simulink model "case9"  (R2024b)
settings: Solver=FixedStepAuto  StartTime=0  StopTime=1  FixedStep=1e-7  RelTol=1e-3
values from neighbouring files (symbols this model uses):
  SG_D_1_D = 0.01056    [IEEE9_case_parameters.m]    (also in case1_parameters.m; case2_parameters.m; case3_parameters.m; case4_parameters.m)
  SG_D_1_EnableSaturation = 0    [IEEE9_case_parameters.m]    (also in case1_parameters.m; case2_parameters.m; case3_parameters.m; case4_parameters.m)
  SG_D_1_f0 = 60    [IEEE9_case_parameters.m]    (also in case1_parameters.m; case2_parameters.m; case3_parameters.m; case4_parameters.m)
  SG_D_1_H = 7.5    [IEEE9_case_parameters.m]    (also in case1_parameters.m; case2_parameters.m; case3_parameters.m; case4_parameters.m)
  SG_D_1_K_A = 20    [IEEE9_case_parameters.m]    (also in case1_parameters.m; case2_parameters.m; case3_parameters.m; case4_parameters.m)
  SG_D_1_K_E = 1.000000e+1    (= 10)    [IEEE9_case_parameters.m]    (also in case1_parameters.m; case2_parameters.m; case3_parameters.m; case4_parameters.m)
  SG_D_1_K_F = 2.363    [IEEE9_case_parameters.m]    (also in case1_parameters.m; case2_parameters.m; case3_parameters.m; case4_parameters.m)
  SG_D_1_K_s = 0.5    [IEEE9_case_parameters.m]    (also in case1_parameters.m = 5; case2_parameters.m = 5; case3_parameters.m = 5; case4_parameters.m = 5)
  SG_D_1_R_a = 0.001088    [IEEE9_case_parameters.m]    (also in case1_parameters.m; case2_parameters.m; case3_parameters.m; case4_parameters.m)
  SG_D_1_S_A = 1    [IEEE9_case_parameters.m]    (also in case1_parameters.m; case2_parameters.m; case3_parameters.m; case4_parameters.m)
  SG_D_1_S_B = 0.103    [IEEE9_case_parameters.m]    (also in case1_parameters.m; case2_parameters.m; case3_parameters.m; case4_parameters.m)
  SG_D_1_S_N = 10.659857    [IEEE9_case_parameters.m]    (also in case1_parameters.m; case2_parameters.m; case3_parameters.m; case4_parameters.m)
  SG_D_1_SpeedPara = 200    [IEEE9_case_parameters.m]    (also in case1_parameters.m; case2_parameters.m; case3_parameters.m; case4_parameters.m)
  SG_D_1_T_0 = 0.720173    [IEEE9_case_parameters.m]    (also in case1_parameters.m = 0.755522; case2_parameters.m = 0.808931; case3_parameters.m = 0.869402; case4_parameters.m = 0.729316)
  SG_D_1_T_1 = 0.3    [IEEE9_case_parameters.m]    (also in case1_parameters.m; case2_parameters.m; case3_parameters.m; case4_parameters.m)
  SG_D_1_T_2 = 0.05    [IEEE9_case_parameters.m]    (also in case1_parameters.m; case2_parameters.m; case3_parameters.m; case4_parameters.m)
  SG_D_1_T_3 = 0.02    [IEEE9_case_parameters.m]    (also in case1_parameters.m; case2_parameters.m; case3_parameters.m; case4_parameters.m)
  SG_D_1_T_4 = 0.005    [IEEE9_case_parameters.m]    (also in case1_parameters.m; case2_parameters.m; case3_parameters.m; case4_parameters.m)
  SG_D_1_T_A = 0.02    [IEEE9_case_parameters.m]    (also in case1_parameters.m; case2_parameters.m; case3_parameters.m; case4_parameters.m)
  SG_D_1_T_dd = 8.000000e+0    (= 8)    [IEEE9_case_parameters.m]    (also in case1_parameters.m; case2_parameters.m; case3_parameters.m; case4_parameters.m)
  SG_D_1_T_ddd = 0.04    [IEEE9_case_parameters.m]    (also in case1_parameters.m; case2_parameters.m; case3_parameters.m; case4_parameters.m)
  SG_D_1_T_E = 0.314    [IEEE9_case_parameters.m]    (also in case1_parameters.m; case2_parameters.m; case3_parameters.m; case4_parameters.m)
  SG_D_1_T_F = 0.35    [IEEE9_case_parameters.m]    (also in case1_parameters.m; case2_parameters.m; case3_parameters.m; case4_parameters.m)
  SG_D_1_T_qd = 0.8    [IEEE9_case_parameters.m]    (also in case1_parameters.m; case2_parameters.m; case3_parameters.m; case4_parameters.m)
  SG_D_1_T_qdd = 0.02    [IEEE9_case_parameters.m]    (also in case1_parameters.m; case2_parameters.m; case3_parameters.m; case4_parameters.m)
  SG_D_1_T_speed = 0.1    [IEEE9_case_parameters.m]    (also in case1_parameters.m = 200; case2_parameters.m = 200; case3_parameters.m = 200; case4_parameters.m = 200)
  SG_D_1_T_w = 0.5    [IEEE9_case_parameters.m]    (also in case1_parameters.m; case2_parameters.m; case3_parameters.m; case4_parameters.m)
  SG_D_1_V_ref = 1.990276    [IEEE9_case_parameters.m]    (also in case1_parameters.m = 2.042296; case2_parameters.m = 2.051388; case3_parameters.m = 2.089584; case4_parameters.m = 2.01845)
  SG_D_1_w_ref = 376.991118    [IEEE9_case_parameters.m]    (also in case1_parameters.m; case2_parameters.m; case3_parameters.m; case4_parameters.m)
  SG_D_1_wb = 6.000000e+1    (= 60)    [IEEE9_case_parameters.m]    (also in case1_parameters.m; case2_parameters.m; case3_parameters.m; case4_parameters.m)
  SG_D_1_x_d = 1.9    [IEEE9_case_parameters.m]    (also in case1_parameters.m; case2_parameters.m; case3_parameters.m; case4_parameters.m)
  SG_D_1_x_dd = 0.302    [IEEE9_case_parameters.m]    (also in case1_parameters.m; case2_parameters.m; case3_parameters.m; case4_parameters.m)
  SG_D_1_x_ddd = 0.204    [IEEE9_case_parameters.m]    (also in case1_parameters.m; case2_parameters.m; case3_parameters.m; case4_parameters.m)
  SG_D_1_x_l = 0.05    [IEEE9_case_parameters.m]    (also in case1_parameters.m; case2_parameters.m; case3_parameters.m; case4_parameters.m)
  SG_D_1_x_q = 1.3    [IEEE9_case_parameters.m]    (also in case1_parameters.m; case2_parameters.m; case3_parameters.m; case4_parameters.m)
  SG_D_1_x_qd = 0.5    [IEEE9_case_parameters.m]    (also in case1_parameters.m; case2_parameters.m; case3_parameters.m; case4_parameters.m)
  SG_D_1_x_qdd = 0.3    [IEEE9_case_parameters.m]    (also in case1_parameters.m; case2_parameters.m; case3_parameters.m; case4_parameters.m)
  SG_D_2_D = 0.02    [IEEE9_case_parameters.m]    (also in case1_parameters.m; case2_parameters.m; case3_parameters.m; case4_parameters.m)
  SG_D_2_EnableSaturation = 0    [IEEE9_case_parameters.m]    (also in case1_parameters.m; case2_parameters.m; case3_parameters.m; case4_parameters.m)
  SG_D_2_f0 = 60    [IEEE9_case_parameters.m]    (also in case1_parameters.m; case2_parameters.m; case3_parameters.m; case4_parameters.m)
  SG_D_2_H = 8.000000e+0    (= 8)    [IEEE9_case_parameters.m]    (also in case1_parameters.m; case2_parameters.m; case3_parameters.m; case4_parameters.m)
  SG_D_2_K_A = 20    [IEEE9_case_parameters.m]    (also in case1_parameters.m; case2_parameters.m; case3_parameters.m; case4_parameters.m)
  SG_D_2_K_E = 1.000000e+1    (= 10)    [IEEE9_case_parameters.m]    (also in case1_parameters.m; case2_parameters.m; case3_parameters.m; case4_parameters.m)
  SG_D_2_K_F = 2.363    [IEEE9_case_parameters.m]    (also in case1_parameters.m; case2_parameters.m; case3_parameters.m; case4_parameters.m)
  SG_D_2_K_s = 0.5    [IEEE9_case_parameters.m]    (also in case1_parameters.m = 4; case2_parameters.m = 4; case3_parameters.m = 4; case4_parameters.m = 4)
  SG_D_2_R_a = 0.001088    [IEEE9_case_parameters.m]    (also in case1_parameters.m; case2_parameters.m; case3_parameters.m; case4_parameters.m)
  SG_D_2_S_A = 1    [IEEE9_case_parameters.m]    (also in case1_parameters.m; case2_parameters.m; case3_parameters.m; case4_parameters.m)
  SG_D_2_S_B = 0.103    [IEEE9_case_parameters.m]    (also in case1_parameters.m; case2_parameters.m; case3_parameters.m; case4_parameters.m)
  SG_D_2_S_N = 10.659857    [IEEE9_case_parameters.m]    (also in case1_parameters.m; case2_parameters.m; case3_parameters.m; case4_parameters.m)
  SG_D_2_SpeedPara = 200    [IEEE9_case_parameters.m]    (also in case1_parameters.m; case2_parameters.m; case3_parameters.m; case4_parameters.m)
  SG_D_2_T_0 = 1.632913    [IEEE9_case_parameters.m]    (also in case1_parameters.m = 1.632925; case2_parameters.m = 1.632915; case3_parameters.m = 1.632914; case4_parameters.m = 1.632927)
  SG_D_2_T_1 = 0.2    [IEEE9_case_parameters.m]    (also in case1_parameters.m; case2_parameters.m; case3_parameters.m; case4_parameters.m)
  SG_D_2_T_2 = 0.05    [IEEE9_case_parameters.m]    (also in case1_parameters.m; case2_parameters.m; case3_parameters.m; case4_parameters.m)
  SG_D_2_T_3 = 0.02    [IEEE9_case_parameters.m]    (also in case1_parameters.m; case2_parameters.m; case3_parameters.m; case4_parameters.m)
  SG_D_2_T_4 = 0.005    [IEEE9_case_parameters.m]    (also in case1_parameters.m; case2_parameters.m; case3_parameters.m; case4_parameters.m)
  SG_D_2_T_A = 0.02    [IEEE9_case_parameters.m]    (also in case1_parameters.m; case2_parameters.m; case3_parameters.m; case4_parameters.m)
  SG_D_2_T_dd = 7.9    [IEEE9_case_parameters.m]    (also in case1_parameters.m; case2_parameters.m; case3_parameters.m; case4_parameters.m)
  SG_D_2_T_ddd = 0.04    [IEEE9_case_parameters.m]    (also in case1_parameters.m; case2_parameters.m; case3_parameters.m; case4_parameters.m)
  SG_D_2_T_E = 0.314    [IEEE9_case_parameters.m]    (also in case1_parameters.m; case2_parameters.m; case3_parameters.m; case4_parameters.m)
  SG_D_2_T_F = 0.35    [IEEE9_case_parameters.m]    (also in case1_parameters.m; case2_parameters.m; case3_parameters.m; case4_parameters.m)
  SG_D_2_T_qd = 0.8    [IEEE9_case_parameters.m]    (also in case1_parameters.m; case2_parameters.m; case3_parameters.m; case4_parameters.m)
  SG_D_2_T_qdd = 0.015    [IEEE9_case_parameters.m]    (also in case1_parameters.m; case2_parameters.m; case3_parameters.m; case4_parameters.m)
  SG_D_2_T_speed = 0.1    [IEEE9_case_parameters.m]    (also in case1_parameters.m = 150; case2_parameters.m = 150; case3_parameters.m = 150; case4_parameters.m = 150)
  SG_D_2_T_w = 0.35    [IEEE9_case_parameters.m]    (also in case1_parameters.m; case2_parameters.m; case3_parameters.m; case4_parameters.m)
  SG_D_2_V_ref = 2.58547    [IEEE9_case_parameters.m]    (also in case1_parameters.m = 2.597896; case2_parameters.m = 2.587136; case3_parameters.m = 2.586042; case4_parameters.m = 2.599679)
  SG_D_2_w_ref = 376.991118    [IEEE9_case_parameters.m]    (also in case1_parameters.m; case2_parameters.m; case3_parameters.m; case4_parameters.m)
  SG_D_2_wb = 6.000000e+1    (= 60)    [IEEE9_case_parameters.m]    (also in case1_parameters.m; case2_parameters.m; case3_parameters.m; case4_parameters.m)
  SG_D_2_x_d = 1.8    [IEEE9_case_parameters.m]    (also in case1_parameters.m; case2_parameters.m; case3_parameters.m; case4_parameters.m)
  SG_D_2_x_dd = 0.302    [IEEE9_case_parameters.m]    (also in case1_parameters.m; case2_parameters.m; case3_parameters.m; case4_parameters.m)
  SG_D_2_x_ddd = 0.204    [IEEE9_case_parameters.m]    (also in case1_parameters.m; case2_parameters.m; case3_parameters.m; case4_parameters.m)
  SG_D_2_x_l = 0.05    [IEEE9_case_parameters.m]    (also in case1_parameters.m; case2_parameters.m; case3_parameters.m; case4_parameters.m)
  SG_D_2_x_q = 1.25    [IEEE9_case_parameters.m]    (also in case1_parameters.m; case2_parameters.m; case3_parameters.m; case4_parameters.m)
  SG_D_2_x_qd = 0.5    [IEEE9_case_parameters.m]    (also in case1_parameters.m; case2_parameters.m; case3_parameters.m; case4_parameters.m)
  SG_D_2_x_qdd = 0.3    [IEEE9_case_parameters.m]    (also in case1_parameters.m; case2_parameters.m; case3_parameters.m; case4_parameters.m)
  SG_D_3_D = 0.02    [IEEE9_case_parameters.m]    (also in case1_parameters.m; case2_parameters.m; case3_parameters.m; case4_parameters.m)
  SG_D_3_EnableSaturation = 0    [IEEE9_case_parameters.m]    (also in case1_parameters.m; case2_parameters.m; case3_parameters.m; case4_parameters.m)
  SG_D_3_f0 = 60    [IEEE9_case_parameters.m]    (also in case1_parameters.m; case2_parameters.m; case3_parameters.m; case4_parameters.m)
  SG_D_3_H = 7.7    [IEEE9_case_parameters.m]    (also in case1_parameters.m; case2_parameters.m; case3_parameters.m; case4_parameters.m)
  SG_D_3_K_A = 20    [IEEE9_case_parameters.m]    (also in case1_parameters.m; case2_parameters.m; case3_parameters.m; case4_parameters.m)
  SG_D_3_K_E = 1.000000e+1    (= 10)    [IEEE9_case_parameters.m]    (also in case1_parameters.m; case2_parameters.m; case3_parameters.m; case4_parameters.m)
  SG_D_3_K_F = 2.363    [IEEE9_case_parameters.m]    (also in case1_parameters.m; case2_parameters.m; case3_parameters.m; case4_parameters.m)
  SG_D_3_K_s = 0.2    [IEEE9_case_parameters.m]    (also in case1_parameters.m = 2; case2_parameters.m = 2; case3_parameters.m = 2; case4_parameters.m = 2)
  SG_D_3_R_a = 0.001088    [IEEE9_case_parameters.m]    (also in case1_parameters.m; case2_parameters.m; case3_parameters.m; case4_parameters.m)
  SG_D_3_S_A = 1    [IEEE9_case_parameters.m]    (also in case1_parameters.m; case2_parameters.m; case3_parameters.m; case4_parameters.m)
  SG_D_3_S_B = 0.103    [IEEE9_case_parameters.m]    (also in case1_parameters.m; case2_parameters.m; case3_parameters.m; case4_parameters.m)
  SG_D_3_S_N = 10.659857    [IEEE9_case_parameters.m]    (also in case1_parameters.m; case2_parameters.m; case3_parameters.m; case4_parameters.m)
  SG_D_3_SpeedPara = 200    [IEEE9_case_parameters.m]    (also in case1_parameters.m; case2_parameters.m; case3_parameters.m; case4_parameters.m)
  SG_D_3_T_0 = 0.850788    [IEEE9_case_parameters.m]    (also in case1_parameters.m = 0.850786; case2_parameters.m = 0.850787; case3_parameters.m; case4_parameters.m = 0.850786)
  SG_D_3_T_1 = 0.2    [IEEE9_case_parameters.m]    (also in case1_parameters.m; case2_parameters.m; case3_parameters.m; case4_parameters.m)
  SG_D_3_T_2 = 0.05    [IEEE9_case_parameters.m]    (also in case1_parameters.m; case2_parameters.m; case3_parameters.m; case4_parameters.m)
  SG_D_3_T_3 = 0.02    [IEEE9_case_parameters.m]    (also in case1_parameters.m; case2_parameters.m; case3_parameters.m; case4_parameters.m)
  SG_D_3_T_4 = 0.005    [IEEE9_case_parameters.m]    (also in case1_parameters.m; case2_parameters.m; case3_parameters.m; case4_parameters.m)
  SG_D_3_T_A = 0.02    [IEEE9_case_parameters.m]    (also in case1_parameters.m; case2_parameters.m; case3_parameters.m; case4_parameters.m)
  SG_D_3_T_dd = 8.1    [IEEE9_case_parameters.m]    (also in case1_parameters.m; case2_parameters.m; case3_parameters.m; case4_parameters.m)
  SG_D_3_T_ddd = 0.04    [IEEE9_case_parameters.m]    (also in case1_parameters.m; case2_parameters.m; case3_parameters.m; case4_parameters.m)
  SG_D_3_T_E = 0.314    [IEEE9_case_parameters.m]    (also in case1_parameters.m; case2_parameters.m; case3_parameters.m; case4_parameters.m)
  SG_D_3_T_F = 0.35    [IEEE9_case_parameters.m]    (also in case1_parameters.m; case2_parameters.m; case3_parameters.m; case4_parameters.m)
  SG_D_3_T_qd = 0.8    [IEEE9_case_parameters.m]    (also in case1_parameters.m; case2_parameters.m; case3_parameters.m; case4_parameters.m)
  SG_D_3_T_qdd = 0.015    [IEEE9_case_parameters.m]    (also in case1_parameters.m; case2_parameters.m; case3_parameters.m; case4_parameters.m)
  SG_D_3_T_speed = 0.1    [IEEE9_case_parameters.m]    (also in case1_parameters.m = 180; case2_parameters.m = 180; case3_parameters.m = 180; case4_parameters.m = 180)
  SG_D_3_T_w = 0.4    [IEEE9_case_parameters.m]    (also in case1_parameters.m; case2_parameters.m; case3_parameters.m; case4_parameters.m)
  SG_D_3_V_ref = 1.892727    [IEEE9_case_parameters.m]    (also in case1_parameters.m = 1.906439; case2_parameters.m = 1.895535; case3_parameters.m = 1.892105; case4_parameters.m = 1.906598)
  SG_D_3_w_ref = 376.991118    [IEEE9_case_parameters.m]    (also in case1_parameters.m; case2_parameters.m; case3_parameters.m; case4_parameters.m)
  SG_D_3_wb = 6.000000e+1    (= 60)    [IEEE9_case_parameters.m]    (also in case1_parameters.m; case2_parameters.m; case3_parameters.m; case4_parameters.m)
  SG_D_3_x_d = 1.85    [IEEE9_case_parameters.m]    (also in case1_parameters.m; case2_parameters.m; case3_parameters.m; case4_parameters.m)
  SG_D_3_x_dd = 0.302    [IEEE9_case_parameters.m]    (also in case1_parameters.m; case2_parameters.m; case3_parameters.m; case4_parameters.m)
  SG_D_3_x_ddd = 0.204    [IEEE9_case_parameters.m]    (also in case1_parameters.m; case2_parameters.m; case3_parameters.m; case4_parameters.m)
  SG_D_3_x_l = 0.05    [IEEE9_case_parameters.m]    (also in case1_parameters.m; case2_parameters.m; case3_parameters.m; case4_parameters.m)
  SG_D_3_x_q = 1.2    [IEEE9_case_parameters.m]    (also in case1_parameters.m; case2_parameters.m; case3_parameters.m; case4_parameters.m)
  SG_D_3_x_qd = 0.5    [IEEE9_case_parameters.m]    (also in case1_parameters.m; case2_parameters.m; case3_parameters.m; case4_parameters.m)
  SG_D_3_x_qdd = 0.3    [IEEE9_case_parameters.m]    (also in case1_parameters.m; case2_parameters.m; case3_parameters.m; case4_parameters.m)
(part 10 of 12)

== system case9/Apparatus/SG_D_3/d_R_f_SG_D_3_block ==
  note: d_R_f_SG_D_3 in case9
      | $-\frac{R_{f,\mathrm{SG},D,3}-\frac{E_{\mathrm{fd},\mathrm{SG},D,3}\,K_{F}}{T_{F}}}{T_{F}}$
      | Automatically generated on 2025-10-31 19:35:23 .
  State_E_fd_SG_D_3_d3338 : Inport
  State_R_f_SG_D_3_c793d : Inport  Port=2
  Constant_K_F_f60d5 : Constant  Value=K_F
  Constant_T_F_71048 : Constant  Value=T_F
  Constant_T_F_ce871 : Constant  Value=T_F
  Divide_2852f : Product  Inputs=*/
  Divide_9196c : Product  Inputs=*/
  Product_70c72 : Product
  Subtract_bfe51 : Sum  Inputs=+-
  Blockout_d_R_f_SG_D_3_3dafc : Outport
  wires:
  State_E_fd_SG_D_3_d3338/1 -> Product_70c72/1
  Constant_T_F_ce871/1 -> Divide_9196c/2
  Constant_K_F_f60d5/1 -> Product_70c72/2
  Product_70c72/1 -> Divide_9196c/1
  Divide_9196c/1 -> Subtract_bfe51/1
  State_R_f_SG_D_3_c793d/1 -> Subtract_bfe51/2
  Subtract_bfe51/1 -> Divide_2852f/1
  Constant_T_F_71048/1 -> Divide_2852f/2
  Divide_2852f/1 -> Blockout_d_R_f_SG_D_3_3dafc/1

== system case9/Apparatus/SG_D_3/d_T_m_SG_D_3_block ==
  note: d_T_m_SG_D_3 in case9
      | $-\frac{T_{m,\mathrm{SG},D,3}-T_{0}+\frac{\mathrm{SpeedPara}\,\left(w_{\mathrm{SG},D,3}-w_{\mathrm{ref}}\right)}{2\,f_{0}\,\pi }}{T_{\mathrm{speed}}}$
      | Automatically generated on 2025-10-31 19:35:20 .
  State_w_SG_D_3_6c006 : Inport
  State_T_m_SG_D_3_889e3 : Inport  Port=2
  Add_05352 : Sum
  Add_c118a : Sum
  Constant_-1_665e1 : Constant  Value=-1
  Constant_2.0_9a1eb : Constant  Value=2.0
  Constant_SpeedPara_3d864 : Constant  Value=SpeedPara
  Constant_T_0_d1871 : Constant  Value=T_0
  Constant_T_speed_e621a : Constant  Value=T_speed
  Constant_f0_70c54 : Constant  Value=f0
  Constant_pi_4d991 : Constant  Value=pi
  Constant_w_ref_62e28 : Constant  Value=w_ref
  Divide_248c6 : Product  Inputs=*/
  Divide_c7cc2 : Product  Inputs=*/
  Product_435bd : Product
  Product_930ed : Product
  Product_9c6c0 : Product
  Product_c4671 : Product
  Subtract_aed96 : Sum  Inputs=+-
  Blockout_d_T_m_SG_D_3_c99ea : Outport
  wires:
  Constant_SpeedPara_3d864/1 -> Product_c4671/1
  Constant_-1_665e1/1 -> Product_9c6c0/1
  Constant_w_ref_62e28/1 -> Add_c118a/2
  State_w_SG_D_3_6c006/1 -> Product_9c6c0/2
  Constant_2.0_9a1eb/1 -> Product_435bd/1
  Product_9c6c0/1 -> Add_c118a/1
  Constant_pi_4d991/1 -> Product_435bd/2
  Add_c118a/1 -> Product_c4671/2
  Product_435bd/1 -> Product_930ed/1
  Constant_f0_70c54/1 -> Product_930ed/2
  Product_c4671/1 -> Divide_c7cc2/1
  Product_930ed/1 -> Divide_c7cc2/2
  Divide_c7cc2/1 -> Add_05352/1
  Constant_T_0_d1871/1 -> Add_05352/2
  Add_05352/1 -> Subtract_aed96/1
  State_T_m_SG_D_3_889e3/1 -> Subtract_aed96/2
  Subtract_aed96/1 -> Divide_248c6/1
  Constant_T_speed_e621a/1 -> Divide_248c6/2
  Divide_248c6/1 -> Blockout_d_T_m_SG_D_3_c99ea/1

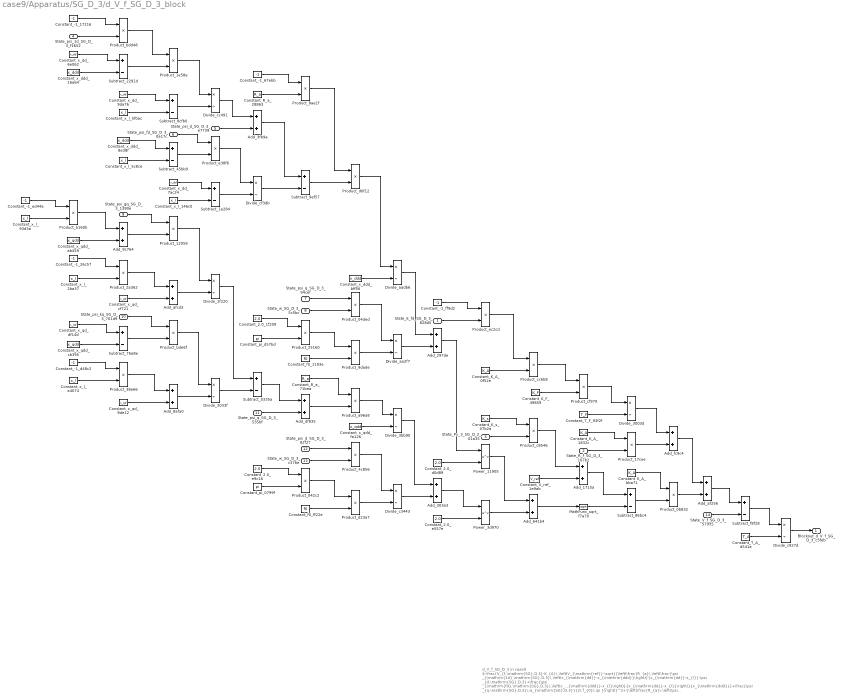
== system case9/Apparatus/SG_D_3/d_V_f_SG_D_3_block ==
  note: d_V_f_SG_D_3 in case9
      | $-\frac{V_{f,\mathrm{SG},D,3}-K_{A}\,\left(V_{\mathrm{ref}}-\sqrt{{\left(\frac{R_{a}\,\left(\frac{\psi _{\mathrm{1d},\mathrm{SG},D,3}\,\left(x_{\mathrm{dd}}-x_{\mathrm{ddd}}\right)}{x_{\mathrm{dd}}-x_{l}}-\psi _{d,\mathrm{SG},D,3}+\frac{\psi _{\mathrm{fd},\mathrm{SG},D,3}\,\left(x_{\mathrm{ddd}}-x_{l}\right)}{x_{\mathrm{dd}}-x_{l}}\right)}{x_{\mathrm{ddd}}}+\frac{\psi _{q,\mathrm{SG},D,3}\,w_{\mathrm{SG},D,3}}{2\,f_{0}\,\pi }\right)}^2+{\left(\frac{R_{a}\,\left(\psi _{q,\mathrm{SG},D,3}+\frac{\psi _{\mathrm{gq},\mathrm{SG},D,3}\,\left(x_{l}-x_{\mathrm{qdd}}\right)}{x_{l}-x_{\mathrm{qd}}}+\frac{\psi _{\mathrm{kq},\mathrm{SG},D,3}\,\left(x_{\mathrm{qd}}-x_{\mathrm{qdd}}\right)}{x_{l}-x_{\mathrm{qd}}}\right)}{x_{\mathrm{qdd}}}+\frac{\psi _{d,\mathrm{SG},D,3}\,w_{\mathrm{SG},D,3}}{2\,f_{0}\,\pi }\right)}^2}+K_{s}\,\mathrm{Px}_{3,\mathrm{SG},D,3}\right)-K_{A}\,R_{f,\mathrm{SG},D,3}+\frac{E_{\mathrm{fd},\mathrm{SG},D,3}\,K_{A}\,K_{F}}{T_{F}}}{T_{A}}$
      | Automatically generated on 2025-10-31 19:35:22 .
  State_E_fd_SG_D_3_828d5 : Inport
  State_R_f_SG_D_3_107b2 : Inport  Port=2
  State_Px_3_SG_D_3_01a35 : Inport  Port=3
  State_psi_1d_SG_D_3_f1652 : Inport  Port=4
  State_psi_d_SG_D_3_e7739 : Inport  Port=5
  State_psi_fd_SG_D_3_0a17c : Inport  Port=6
  State_psi_q_SG_D_3_94cef : Inport  Port=7
  State_w_SG_D_3_5c5bc : Inport  Port=8
  State_psi_gq_SG_D_3_1390e : Inport  Port=9
  State_psi_kq_SG_D_3_701d9 : Inport  Port=10
  State_psi_q_SG_D_3_535bf : Inport  Port=11
  State_psi_d_SG_D_3_82f27 : Inport  Port=12
  State_w_SG_D_3_c376e : Inport  Port=13
  State_V_f_SG_D_3_57935 : Inport  Port=14
  Add_1715a : Sum
  Add_297de : Sum
  Add_303a3 : Sum
  Add_3fb9a : Sum
  Add_641b4 : Sum
  Add_8afa0 : Sum
  Add_9c764 : Sum
  Add_af256 : Sum
  Add_afcd3 : Sum
  Add_df835 : Sum
  Add_fc9c4 : Sum
  Constant_-1_17216 : Constant  Value=-1
  Constant_-1_26c57 : Constant  Value=-1
  Constant_-1_67ebb : Constant  Value=-1
  Constant_-1_d48c2 : Constant  Value=-1
  Constant_-1_ed44a : Constant  Value=-1
  Constant_-1_ff9d2 : Constant  Value=-1
  Constant_2.0_1f209 : Constant  Value=2.0
  Constant_2.0_d0d89 : Constant  Value=2.0
  Constant_2.0_e557e : Constant  Value=2.0
  Constant_2.0_e9c16 : Constant  Value=2.0
  Constant_K_A_0f52e : Constant  Value=K_A
  Constant_K_A_1832c : Constant  Value=K_A
  Constant_K_A_bba71 : Constant  Value=K_A
  Constant_K_F_49859 : Constant  Value=K_F
  Constant_K_s_07b2a : Constant  Value=K_s
  Constant_R_a_28863 : Constant  Value=R_a
  Constant_R_a_71bea : Constant  Value=R_a
  Constant_T_A_d541a : Constant  Value=T_A
  Constant_T_F_93f2f : Constant  Value=T_F
  Constant_V_ref_1e9ab : Constant  Value=V_ref
  Constant_f0_1193e : Constant  Value=f0
  Constant_f0_ff22e : Constant  Value=f0
  Constant_pi_0799f : Constant  Value=pi
  Constant_pi_d57bd : Constant  Value=pi
  Constant_x_dd_6e062 : Constant  Value=x_dd
  Constant_x_dd_7ac24 : Constant  Value=x_dd
  Constant_x_dd_9da76 : Constant  Value=x_dd
  Constant_x_ddd_16a64 : Constant  Value=x_ddd
  Constant_x_ddd_8e38f : Constant  Value=x_ddd
  Constant_x_ddd_bff56 : Constant  Value=x_ddd
  Constant_x_l_146c0 : Constant  Value=x_l
  Constant_x_l_2ba37 : Constant  Value=x_l
  Constant_x_l_5c8ce : Constant  Value=x_l
  Constant_x_l_5f0ac : Constant  Value=x_l
  Constant_x_l_93d3a : Constant  Value=x_l
  Constant_x_l_a4074 : Constant  Value=x_l
  Constant_x_qd_9de12 : Constant  Value=x_qd
  Constant_x_qd_cf721 : Constant  Value=x_qd
  Constant_x_qd_df14d : Constant  Value=x_qd
  Constant_x_qdd_ab459 : Constant  Value=x_qdd
  Constant_x_qdd_cb395 : Constant  Value=x_qdd
  Constant_x_qdd_fa126 : Constant  Value=x_qdd
  Divide_1f220 : Product  Inputs=*/
  Divide_3003d : Product  Inputs=*/
  Divide_3033f : Product  Inputs=*/
  Divide_3bb90 : Product  Inputs=*/
  Divide_aa2f7 : Product  Inputs=*/
  Divide_aadb6 : Product  Inputs=*/
  Divide_c3443 : Product  Inputs=*/
  Divide_c927d : Product  Inputs=*/
  Divide_cc491 : Product  Inputs=*/
  Divide_cf3db : Product  Inputs=*/
  MathFunc_sqrt_f7a70 : Sqrt
  Power_11905 : Math  Operator=pow
  Power_3d970 : Math  Operator=pow
  Product_042c2 : Product
  Product_04ded : Product
  Product_0b832 : Product
  Product_12059 : Product
  Product_17cee : Product
  Product_1e58e : Product
  Product_25160 : Product
  Product_2a362 : Product
  Product_38e66 : Product
  Product_4c856 : Product
  Product_8ae1f : Product
  Product_9dade : Product
  Product_a96a8 : Product
  Product_b160b : Product
  Product_bdd48 : Product
  Product_bde6f : Product
  Product_c8546 : Product
  Product_cc6b8 : Product
  Product_cf970 : Product
  Product_d0f12 : Product
  Product_d23a7 : Product
  Product_e38f6 : Product
  Product_ec2cd : Product
  Subtract_0335a : Sum  Inputs=+-
  Subtract_1e284 : Sum  Inputs=+-
  Subtract_2291d : Sum  Inputs=+-
  Subtract_45bb9 : Sum  Inputs=+-
  Subtract_76a8e : Sum  Inputs=+-
  Subtract_86bc4 : Sum  Inputs=+-
  Subtract_8cfb0 : Sum  Inputs=+-
  Subtract_9ef57 : Sum  Inputs=+-
  Subtract_f8f28 : Sum  Inputs=+-
  Blockout_d_V_f_SG_D_3_c5feb : Outport
  wires:
  Constant_K_A_1832c/1 -> Product_17cee/1
  Constant_-1_ed44a/1 -> Product_b160b/1
  Subtract_45bb9/1 -> Product_e38f6/2
  Constant_x_l_93d3a/1 -> Product_b160b/2
  Divide_c3443/1 -> Add_303a3/2
  Constant_-1_17216/1 -> Product_bdd48/1
  State_psi_1d_SG_D_3_f1652/1 -> Product_bdd48/2
  Constant_x_dd_6e062/1 -> Subtract_2291d/1
  Divide_cf3db/1 -> Subtract_9ef57/2
  Product_b160b/1 -> Add_9c764/1
  Constant_x_qdd_ab459/1 -> Add_9c764/2
  Constant_x_ddd_16a64/1 -> Subtract_2291d/2
  Constant_2.0_e557e/1 -> Power_3d970/2
  Constant_-1_26c57/1 -> Product_2a362/1
  Divide_1f220/1 -> Subtract_0335a/1
  Subtract_8cfb0/1 -> Divide_cc491/2
  Constant_x_l_2ba37/1 -> Product_2a362/2
  Constant_x_qd_df14d/1 -> Subtract_76a8e/1
  State_w_SG_D_3_5c5bc/1 -> Product_04ded/2
  Constant_x_qdd_cb395/1 -> Subtract_76a8e/2
  Constant_2.0_1f209/1 -> Product_25160/1
  Constant_-1_d48c2/1 -> Product_38e66/1
  Constant_pi_d57bd/1 -> Product_25160/2
  Add_3fb9a/1 -> Subtract_9ef57/1
  Constant_x_l_a4074/1 -> Product_38e66/2
  Product_bdd48/1 -> Product_1e58e/1
  Subtract_2291d/1 -> Product_1e58e/2
  Constant_2.0_e9c16/1 -> Product_042c2/1
  Constant_x_dd_9da76/1 -> Subtract_8cfb0/1
  Constant_pi_0799f/1 -> Product_042c2/2
  Constant_x_l_5f0ac/1 -> Subtract_8cfb0/2
  Constant_x_ddd_8e38f/1 -> Subtract_45bb9/1
  Constant_x_l_5c8ce/1 -> Subtract_45bb9/2
  State_psi_gq_SG_D_3_1390e/1 -> Product_12059/1
  Constant_x_l_146c0/1 -> Subtract_1e284/2
  Add_9c764/1 -> Product_12059/2
  Product_2a362/1 -> Add_afcd3/1
  Product_12059/1 -> Divide_1f220/1
  Constant_x_qd_cf721/1 -> Add_afcd3/2
  State_psi_kq_SG_D_3_701d9/1 -> Product_bde6f/1
  State_psi_q_SG_D_3_94cef/1 -> Product_04ded/1
  Add_297de/1 -> Power_11905/1
  Subtract_76a8e/1 -> Product_bde6f/2
  Constant_f0_1193e/1 -> Product_9dade/2
  Product_25160/1 -> Product_9dade/1
  Constant_x_qd_9de12/1 -> Add_8afa0/2
  Product_38e66/1 -> Add_8afa0/1
  Product_1e58e/1 -> Divide_cc491/1
  State_psi_fd_SG_D_3_0a17c/1 -> Product_e38f6/1
  Constant_x_dd_7ac24/1 -> Subtract_1e284/1
  Add_afcd3/1 -> Divide_1f220/2
  Add_641b4/1 -> MathFunc_sqrt_f7a70/1
  Product_bde6f/1 -> Divide_3033f/1
  Add_8afa0/1 -> Divide_3033f/2
  Product_8ae1f/1 -> Product_d0f12/1
  Divide_cc491/1 -> Add_3fb9a/1
  Add_1715a/1 -> Subtract_86bc4/1
  State_psi_d_SG_D_3_e7739/1 -> Add_3fb9a/2
  Product_e38f6/1 -> Divide_cf3db/1
  Subtract_1e284/1 -> Divide_cf3db/2
  MathFunc_sqrt_f7a70/1 -> Subtract_86bc4/2
  Divide_3033f/1 -> Subtract_0335a/2
  Constant_-1_67ebb/1 -> Product_8ae1f/1
  Constant_R_a_28863/1 -> Product_8ae1f/2
  Subtract_0335a/1 -> Add_df835/1
  State_psi_q_SG_D_3_535bf/1 -> Add_df835/2
  Subtract_9ef57/1 -> Product_d0f12/2
  Constant_R_a_71bea/1 -> Product_a96a8/1
  Add_df835/1 -> Product_a96a8/2
  State_psi_d_SG_D_3_82f27/1 -> Product_4c856/1
  State_w_SG_D_3_c376e/1 -> Product_4c856/2
  Product_042c2/1 -> Product_d23a7/1
  Constant_f0_ff22e/1 -> Product_d23a7/2
  Product_d0f12/1 -> Divide_aadb6/1
  Constant_x_ddd_bff56/1 -> Divide_aadb6/2
  Product_04ded/1 -> Divide_aa2f7/1
  Product_9dade/1 -> Divide_aa2f7/2
  Product_a96a8/1 -> Divide_3bb90/1
  Constant_x_qdd_fa126/1 -> Divide_3bb90/2
  Product_4c856/1 -> Divide_c3443/1
  Product_d23a7/1 -> Divide_c3443/2
  Divide_aadb6/1 -> Add_297de/1
  Divide_aa2f7/1 -> Add_297de/2
  Divide_3bb90/1 -> Add_303a3/1
  Constant_-1_ff9d2/1 -> Product_ec2cd/1
  State_E_fd_SG_D_3_828d5/1 -> Product_ec2cd/2
  Constant_2.0_d0d89/1 -> Power_11905/2
  Add_303a3/1 -> Power_3d970/1
  Product_ec2cd/1 -> Product_cc6b8/1
  Constant_K_A_0f52e/1 -> Product_cc6b8/2
  Constant_K_s_07b2a/1 -> Product_c8546/1
  State_Px_3_SG_D_3_01a35/1 -> Product_c8546/2
  Power_11905/1 -> Add_641b4/1
  Power_3d970/1 -> Add_641b4/2
  Product_cc6b8/1 -> Product_cf970/1
  Constant_K_F_49859/1 -> Product_cf970/2
  Product_c8546/1 -> Add_1715a/1
  Constant_V_ref_1e9ab/1 -> Add_1715a/2
  Product_cf970/1 -> Divide_3003d/1
  Constant_T_F_93f2f/1 -> Divide_3003d/2
  Add_af256/1 -> Subtract_f8f28/1
  State_R_f_SG_D_3_107b2/1 -> Product_17cee/2
  Divide_3003d/1 -> Add_fc9c4/1
  Product_17cee/1 -> Add_fc9c4/2
  Constant_K_A_bba71/1 -> Product_0b832/1
  Subtract_86bc4/1 -> Product_0b832/2
  Add_fc9c4/1 -> Add_af256/1
  Product_0b832/1 -> Add_af256/2
  State_V_f_SG_D_3_57935/1 -> Subtract_f8f28/2
  Subtract_f8f28/1 -> Divide_c927d/1
  Constant_T_A_d541a/1 -> Divide_c927d/2
  Divide_c927d/1 -> Blockout_d_V_f_SG_D_3_c5feb/1

== system case9/Apparatus/SG_D_3/d_psi_1d_SG_D_3_block ==
  note: d_psi_1d_SG_D_3 in case9
      | $-\frac{\psi _{\mathrm{1d},\mathrm{SG},D,3}-\psi _{\mathrm{fd},\mathrm{SG},D,3}+\frac{\left(x_{\mathrm{dd}}-x_{l}\right)\,\left(\frac{\psi _{\mathrm{1d},\mathrm{SG},D,3}\,\left(x_{\mathrm{dd}}-x_{\mathrm{ddd}}\right)}{x_{\mathrm{dd}}-x_{l}}-\psi _{d,\mathrm{SG},D,3}+\frac{\psi _{\mathrm{fd},\mathrm{SG},D,3}\,\left(x_{\mathrm{ddd}}-x_{l}\right)}{x_{\mathrm{dd}}-x_{l}}\right)}{x_{\mathrm{ddd}}}}{T_{\mathrm{ddd}}}$
      | Automatically generated on 2025-10-31 19:35:15 .
  State_psi_1d_SG_D_3_f1798 : Inport
  State_psi_fd_SG_D_3_480a9 : Inport  Port=2
  State_psi_1d_SG_D_3_e9e74 : Inport  Port=3
  State_psi_d_SG_D_3_8d7eb : Inport  Port=4
  State_psi_fd_SG_D_3_5e039 : Inport  Port=5
  Add_8f520 : Sum
  Add_cfb63 : Sum
  Add_f27cc : Sum
  Constant_-1_599e5 : Constant  Value=-1
  Constant_-1_ccd31 : Constant  Value=-1
  Constant_T_ddd_aaa23 : Constant  Value=T_ddd
  Constant_x_dd_045d7 : Constant  Value=x_dd
  Constant_x_dd_221c5 : Constant  Value=x_dd
  Constant_x_dd_70220 : Constant  Value=x_dd
  Constant_x_dd_e18f6 : Constant  Value=x_dd
  Constant_x_ddd_61c19 : Constant  Value=x_ddd
  Constant_x_ddd_aa5ef : Constant  Value=x_ddd
  Constant_x_ddd_cfe5c : Constant  Value=x_ddd
  Constant_x_l_1330e : Constant  Value=x_l
  Constant_x_l_6a916 : Constant  Value=x_l
  Constant_x_l_7ef89 : Constant  Value=x_l
  Constant_x_l_d79ee : Constant  Value=x_l
  Divide_1c66d : Product  Inputs=*/
  Divide_3e7d3 : Product  Inputs=*/
  Divide_899c7 : Product  Inputs=*/
  Divide_e8ce5 : Product  Inputs=*/
  Product_32a07 : Product
  Product_752f9 : Product
  Product_ab727 : Product
  Product_db9c4 : Product
  Product_efa34 : Product
  Subtract_06230 : Sum  Inputs=+-
  Subtract_550d6 : Sum  Inputs=+-
  Subtract_89028 : Sum  Inputs=+-
  Subtract_9c560 : Sum  Inputs=+-
  Subtract_c319f : Sum  Inputs=+-
  Subtract_ee8db : Sum  Inputs=+-
  Blockout_d_psi_1d_SG_D_3_29df6 : Outport
  wires:
  Divide_e8ce5/1 -> Add_f27cc/1
  Subtract_06230/1 -> Product_752f9/2
  Constant_-1_599e5/1 -> Product_32a07/1
  Constant_x_dd_045d7/1 -> Subtract_ee8db/1
  State_psi_1d_SG_D_3_e9e74/1 -> Product_32a07/2
  Product_32a07/1 -> Product_752f9/1
  Constant_x_dd_70220/1 -> Subtract_06230/1
  Constant_x_ddd_61c19/1 -> Subtract_06230/2
  Constant_x_l_6a916/1 -> Subtract_ee8db/2
  Constant_x_ddd_aa5ef/1 -> Subtract_c319f/1
  Divide_1c66d/1 -> Blockout_d_psi_1d_SG_D_3_29df6/1
  Constant_x_l_7ef89/1 -> Subtract_c319f/2
  Product_752f9/1 -> Divide_e8ce5/1
  Subtract_ee8db/1 -> Divide_e8ce5/2
  State_psi_fd_SG_D_3_5e039/1 -> Product_db9c4/1
  Subtract_c319f/1 -> Product_db9c4/2
  Constant_x_dd_e18f6/1 -> Subtract_550d6/1
  Constant_x_l_d79ee/1 -> Subtract_550d6/2
  State_psi_d_SG_D_3_8d7eb/1 -> Add_f27cc/2
  Product_db9c4/1 -> Divide_899c7/1
  Subtract_550d6/1 -> Divide_899c7/2
  Constant_x_dd_221c5/1 -> Subtract_9c560/1
  Constant_x_l_1330e/1 -> Subtract_9c560/2
  Add_f27cc/1 -> Subtract_89028/1
  Divide_899c7/1 -> Subtract_89028/2
  Constant_-1_ccd31/1 -> Product_ab727/1
  State_psi_1d_SG_D_3_f1798/1 -> Product_ab727/2
  State_psi_fd_SG_D_3_480a9/1 -> Add_8f520/2
  Subtract_9c560/1 -> Product_efa34/1
  Subtract_89028/1 -> Product_efa34/2
  Product_ab727/1 -> Add_8f520/1
  Product_efa34/1 -> Divide_3e7d3/1
  Constant_x_ddd_cfe5c/1 -> Divide_3e7d3/2
  Add_8f520/1 -> Add_cfb63/1
  Divide_3e7d3/1 -> Add_cfb63/2
  Add_cfb63/1 -> Divide_1c66d/1
  Constant_T_ddd_aaa23/1 -> Divide_1c66d/2

== system case9/Apparatus/SG_D_3/d_psi_d_SG_D_3_block ==
  note: d_psi_d_SG_D_3 in case9
      | $2\,\pi \,f_{0}\,\left(v_{d,\mathrm{SG},D,3}\,\sin\left(\theta _{\mathrm{SG},D,3}\right)-v_{q,\mathrm{SG},D,3}\,\cos\left(\theta _{\mathrm{SG},D,3}\right)+\frac{R_{a}\,\left(\frac{\psi _{\mathrm{1d},\mathrm{SG},D,3}\,\left(x_{\mathrm{dd}}-x_{\mathrm{ddd}}\right)}{x_{\mathrm{dd}}-x_{l}}-\psi _{d,\mathrm{SG},D,3}+\frac{\psi _{\mathrm{fd},\mathrm{SG},D,3}\,\left(x_{\mathrm{ddd}}-x_{l}\right)}{x_{\mathrm{dd}}-x_{l}}\right)}{x_{\mathrm{ddd}}}+\frac{\psi _{q,\mathrm{SG},D,3}\,w_{\mathrm{SG},D,3}}{2\,f_{0}\,\pi }\right)$
      | Automatically generated on 2025-10-31 19:35:12 .
  State_psi_1d_SG_D_3_f6eb2 : Inport
  State_psi_d_SG_D_3_3203c : Inport  Port=2
  State_psi_fd_SG_D_3_4f0f8 : Inport  Port=3
  Input_v_d_SG_D_3_166ca : Inport  Port=4
  State_theta_SG_D_3_1ef30 : Inport  Port=5
  Input_v_q_SG_D_3_f40f1 : Inport  Port=6
  State_theta_SG_D_3_45611 : Inport  Port=7
  State_psi_q_SG_D_3_41010 : Inport  Port=8
  State_w_SG_D_3_31722 : Inport  Port=9
  Add_0b5cf : Sum
  Add_d7a66 : Sum
  Constant_-1_e2908 : Constant  Value=-1
  Constant_-2.0_d1fed : Constant  Value=-2.0
  Constant_2.0_8e3c6 : Constant  Value=2.0
  Constant_R_a_36530 : Constant  Value=R_a
  Constant_f0_06954 : Constant  Value=f0
  Constant_f0_e3908 : Constant  Value=f0
  Constant_pi_81b2d : Constant  Value=pi
  Constant_pi_a1fb9 : Constant  Value=pi
  Constant_x_dd_2f379 : Constant  Value=x_dd
  Constant_x_dd_485b5 : Constant  Value=x_dd
  Constant_x_dd_8116b : Constant  Value=x_dd
  Constant_x_ddd_1c0c0 : Constant  Value=x_ddd
  Constant_x_ddd_b7481 : Constant  Value=x_ddd
  Constant_x_ddd_e9c66 : Constant  Value=x_ddd
  Constant_x_l_45c80 : Constant  Value=x_l
  Constant_x_l_64704 : Constant  Value=x_l
  Constant_x_l_9a9f1 : Constant  Value=x_l
  Divide_28b35 : Product  Inputs=*/
  Divide_98ded : Product  Inputs=*/
  Divide_fa05d : Product  Inputs=*/
  Divide_fe6ef : Product  Inputs=*/
  MathFunc_cos_53092 : Trigonometry  Operator=cos
  MathFunc_sin_823e8 : Trigonometry
  Product_20174 : Product
  Product_28f25 : Product
  Product_29988 : Product
  Product_3ce94 : Product
  Product_510dd : Product
  Product_7cf46 : Product
  Product_89e2e : Product
  Product_a6213 : Product
  Product_c6cd5 : Product
  Product_c8ed2 : Product
  Product_cbae0 : Product
  Product_dfd33 : Product
  Subtract_003a6 : Sum  Inputs=+-
  Subtract_3995b : Sum  Inputs=+-
  Subtract_411fc : Sum  Inputs=+-
  Subtract_790b1 : Sum  Inputs=+-
  Subtract_aadb8 : Sum  Inputs=+-
  Subtract_d1880 : Sum  Inputs=+-
  Subtract_e76f2 : Sum  Inputs=+-
  Blockout_d_psi_d_SG_D_3_06261 : Outport
  wires:
  Constant_-1_e2908/1 -> Product_510dd/1
  Constant_2.0_8e3c6/1 -> Product_cbae0/1
  Constant_x_dd_8116b/1 -> Subtract_d1880/1
  State_psi_1d_SG_D_3_f6eb2/1 -> Product_510dd/2
  Constant_x_dd_2f379/1 -> Subtract_aadb8/1
  Constant_pi_81b2d/1 -> Product_cbae0/2
  Constant_x_ddd_e9c66/1 -> Subtract_d1880/2
  Product_510dd/1 -> Product_20174/1
  Product_cbae0/1 -> Product_a6213/1
  Subtract_d1880/1 -> Product_20174/2
  Constant_-2.0_d1fed/1 -> Product_7cf46/1
  Constant_x_l_45c80/1 -> Subtract_aadb8/2
  Constant_x_ddd_b7481/1 -> Subtract_411fc/1
  Constant_pi_a1fb9/1 -> Product_7cf46/2
  Constant_x_l_64704/1 -> Subtract_411fc/2
  Product_28f25/1 -> Divide_98ded/1
  Product_20174/1 -> Divide_28b35/1
  Subtract_aadb8/1 -> Divide_28b35/2
  State_psi_fd_SG_D_3_4f0f8/1 -> Product_c8ed2/1
  Subtract_411fc/1 -> Product_c8ed2/2
  Constant_x_dd_485b5/1 -> Subtract_e76f2/1
  Constant_x_l_9a9f1/1 -> Subtract_e76f2/2
  Divide_98ded/1 -> Subtract_003a6/2
  Divide_28b35/1 -> Add_d7a66/1
  Subtract_790b1/1 -> Product_c6cd5/2
  State_psi_d_SG_D_3_3203c/1 -> Add_d7a66/2
  Product_c8ed2/1 -> Divide_fe6ef/1
  Subtract_e76f2/1 -> Divide_fe6ef/2
  Add_d7a66/1 -> Subtract_790b1/1
  Divide_fe6ef/1 -> Subtract_790b1/2
  Product_3ce94/1 -> Add_0b5cf/2
  Constant_R_a_36530/1 -> Product_c6cd5/1
  Product_89e2e/1 -> Product_29988/1
  State_theta_SG_D_3_1ef30/1 -> MathFunc_sin_823e8/1
  Product_c6cd5/1 -> Divide_fa05d/1
  Constant_x_ddd_1c0c0/1 -> Divide_fa05d/2
  Input_v_d_SG_D_3_166ca/1 -> Product_dfd33/1
  State_w_SG_D_3_31722/1 -> Product_28f25/2
  MathFunc_sin_823e8/1 -> Product_dfd33/2
  State_theta_SG_D_3_45611/1 -> MathFunc_cos_53092/1
  MathFunc_cos_53092/1 -> Product_3ce94/2
  Divide_fa05d/1 -> Subtract_3995b/1
  Product_dfd33/1 -> Subtract_3995b/2
  Input_v_q_SG_D_3_f40f1/1 -> Product_3ce94/1
  State_psi_q_SG_D_3_41010/1 -> Product_28f25/1
  Constant_f0_e3908/1 -> Product_a6213/2
  Subtract_3995b/1 -> Add_0b5cf/1
  Product_a6213/1 -> Divide_98ded/2
  Product_7cf46/1 -> Product_89e2e/1
  Constant_f0_06954/1 -> Product_89e2e/2
  Add_0b5cf/1 -> Subtract_003a6/1
  Subtract_003a6/1 -> Product_29988/2
  Product_29988/1 -> Blockout_d_psi_d_SG_D_3_06261/1

== system case9/Apparatus/SG_D_3/d_psi_fd_SG_D_3_block ==
  note: d_psi_fd_SG_D_3 in case9
      | $-\frac{\psi _{\mathrm{fd},\mathrm{SG},D,3}-E_{\mathrm{fd},\mathrm{SG},D,3}+\left(x_{d}-x_{\mathrm{dd}}\right)\,\left(\frac{\frac{\psi _{\mathrm{1d},\mathrm{SG},D,3}\,\left(x_{\mathrm{dd}}-x_{\mathrm{ddd}}\right)}{x_{\mathrm{dd}}-x_{l}}-\psi _{d,\mathrm{SG},D,3}+\frac{\psi _{\mathrm{fd},\mathrm{SG},D,3}\,\left(x_{\mathrm{ddd}}-x_{l}\right)}{x_{\mathrm{dd}}-x_{l}}}{x_{\mathrm{ddd}}}-\frac{\left(x_{\mathrm{dd}}-x_{\mathrm{ddd}}\right)\,\left(\psi _{\mathrm{1d},\mathrm{SG},D,3}-\psi _{\mathrm{fd},\mathrm{SG},D,3}+\frac{\left(x_{\mathrm{dd}}-x_{l}\right)\,\left(\frac{\psi _{\mathrm{1d},\mathrm{SG},D,3}\,\left(x_{\mathrm{dd}}-x_{\mathrm{ddd}}\right)}{x_{\mathrm{dd}}-x_{l}}-\psi _{d,\mathrm{SG},D,3}+\frac{\psi _{\mathrm{fd},\mathrm{SG},D,3}\,\left(x_{\mathrm{ddd}}-x_{l}\right)}{x_{\mathrm{dd}}-x_{l}}\right)}{x_{\mathrm{ddd}}}\right)}{{\left(x_{\mathrm{dd}}-x_{l}\right)}^2}\right)}{T_{\mathrm{dd}}}$
      | Automatically generated on 2025-10-31 19:35:15 .
  State_E_fd_SG_D_3_c4807 : Inport
  State_psi_fd_SG_D_3_a0d97 : Inport  Port=2
  State_psi_1d_SG_D_3_83346 : Inport  Port=3
  State_psi_fd_SG_D_3_748b1 : Inport  Port=4
  State_psi_1d_SG_D_3_b7a7b : Inport  Port=5
  State_psi_d_SG_D_3_89a39 : Inport  Port=6
  State_psi_fd_SG_D_3_e2a77 : Inport  Port=7
  State_psi_1d_SG_D_3_a323d : Inport  Port=8
  State_psi_d_SG_D_3_2010b : Inport  Port=9
  State_psi_fd_SG_D_3_3a0d7 : Inport  Port=10
  Add_a5e84 : Sum
  Add_c0b37 : Sum
  Constant_-1_27e1c : Constant  Value=-1
  Constant_-1_c4220 : Constant  Value=-1
  Constant_-1_c8b9d : Constant  Value=-1
  Constant_2.0_c8f6e : Constant  Value=2.0
  Constant_T_dd_bc5d2 : Constant  Value=T_dd
  Constant_x_d_61565 : Constant  Value=x_d
  Constant_x_dd_2166e : Constant  Value=x_dd
  Constant_x_dd_57478 : Constant  Value=x_dd
  Constant_x_dd_60261 : Constant  Value=x_dd
  Constant_x_dd_81e98 : Constant  Value=x_dd
  Constant_x_dd_8670c : Constant  Value=x_dd
  Constant_x_dd_c53f4 : Constant  Value=x_dd
  Constant_x_dd_c59a0 : Constant  Value=x_dd
  Constant_x_dd_d93a4 : Constant  Value=x_dd
  Constant_x_dd_e6636 : Constant  Value=x_dd
  Constant_x_dd_f6e51 : Constant  Value=x_dd
  Constant_x_ddd_0c764 : Constant  Value=x_ddd
  Constant_x_ddd_24bf1 : Constant  Value=x_ddd
  Constant_x_ddd_64f4b : Constant  Value=x_ddd
  Constant_x_ddd_83299 : Constant  Value=x_ddd
  Constant_x_ddd_debb3 : Constant  Value=x_ddd
  Constant_x_ddd_deeeb : Constant  Value=x_ddd
  Constant_x_ddd_fc852 : Constant  Value=x_ddd
  Constant_x_l_01786 : Constant  Value=x_l
  Constant_x_l_16664 : Constant  Value=x_l
  Constant_x_l_40a10 : Constant  Value=x_l
  Constant_x_l_4c4de : Constant  Value=x_l
  Constant_x_l_6c4a6 : Constant  Value=x_l
  Constant_x_l_6f3da : Constant  Value=x_l
  Constant_x_l_81e97 : Constant  Value=x_l
  Constant_x_l_c0c62 : Constant  Value=x_l
  Divide_18b4f : Product  Inputs=*/
  Divide_19a64 : Product  Inputs=*/
  Divide_23144 : Product  Inputs=*/
  Divide_4a71c : Product  Inputs=*/
  Divide_55e59 : Product  Inputs=*/
  Divide_b486e : Product  Inputs=*/
  Divide_ce65d : Product  Inputs=*/
  Divide_d1f36 : Product  Inputs=*/
  Power_622e4 : Math  Operator=pow
  Product_1c2f3 : Product
  Product_27e1f : Product
  Product_30c76 : Product
  Product_7164e : Product
  Product_75d1c : Product
  Product_76ec5 : Product
  Product_8e9e1 : Product
  Product_8fa56 : Product
  Product_b3298 : Product
  Product_eaf90 : Product
  Subtract_06353 : Sum  Inputs=+-
  Subtract_0a74c : Sum  Inputs=+-
  Subtract_0d45b : Sum  Inputs=+-
  Subtract_178f7 : Sum  Inputs=+-
  Subtract_2e1b6 : Sum  Inputs=+-
  Subtract_45bc0 : Sum  Inputs=+-
  Subtract_48db2 : Sum  Inputs=+-
  Subtract_49ce1 : Sum  Inputs=+-
  Subtract_89049 : Sum  Inputs=+-
  Subtract_8fd09 : Sum  Inputs=+-
  Subtract_9ff2b : Sum  Inputs=+-
  Subtract_aa4e5 : Sum  Inputs=+-
  Subtract_c63d1 : Sum  Inputs=+-
  Subtract_c7762 : Sum  Inputs=+-
  Subtract_ceb76 : Sum  Inputs=+-
  Subtract_d5f20 : Sum  Inputs=+-
  Subtract_e3c67 : Sum  Inputs=+-
  Subtract_eae77 : Sum  Inputs=+-
  Subtract_ec1ee : Sum  Inputs=+-
  Blockout_d_psi_fd_SG_D_3_350b8 : Outport
  wires:
  Product_76ec5/1 -> Divide_23144/1
  Constant_-1_c8b9d/1 -> Product_8fa56/1
  Subtract_2e1b6/1 -> Product_27e1f/2
  State_psi_1d_SG_D_3_b7a7b/1 -> Product_8fa56/2
  Constant_x_l_01786/1 -> Subtract_45bc0/2
  Constant_x_dd_81e98/1 -> Subtract_2e1b6/1
  Constant_x_ddd_fc852/1 -> Subtract_2e1b6/2
  Product_8fa56/1 -> Product_27e1f/1
  Constant_x_dd_d93a4/1 -> Subtract_e3c67/1
  Constant_x_l_6c4a6/1 -> Subtract_e3c67/2
  Constant_x_ddd_83299/1 -> Subtract_eae77/2
  Constant_x_ddd_0c764/1 -> Subtract_8fd09/1
  Constant_x_l_40a10/1 -> Subtract_8fd09/2
  Product_75d1c/1 -> Product_b3298/1
  Product_27e1f/1 -> Divide_b486e/1
  Subtract_e3c67/1 -> Divide_b486e/2
  State_psi_fd_SG_D_3_e2a77/1 -> Product_8e9e1/1
  Constant_x_ddd_64f4b/1 -> Subtract_45bc0/1
  Subtract_8fd09/1 -> Product_8e9e1/2
  Constant_x_dd_8670c/1 -> Subtract_0a74c/1
  Constant_-1_c4220/1 -> Product_75d1c/1
  Constant_x_l_6f3da/1 -> Subtract_0a74c/2
  Product_b3298/1 -> Divide_19a64/1
  Divide_b486e/1 -> Add_c0b37/1
  Product_1c2f3/1 -> Divide_ce65d/1
  State_psi_d_SG_D_3_89a39/1 -> Add_c0b37/2
  State_psi_fd_SG_D_3_3a0d7/1 -> Product_1c2f3/1
  Product_8e9e1/1 -> Divide_4a71c/1
  Constant_x_dd_c53f4/1 -> Subtract_178f7/1
  Subtract_0a74c/1 -> Divide_4a71c/2
  Constant_x_l_4c4de/1 -> Subtract_d5f20/2
  Constant_x_dd_57478/1 -> Subtract_c7762/1
  Subtract_0d45b/1 -> Product_eaf90/2
  Constant_x_l_c0c62/1 -> Subtract_c7762/2
  Divide_19a64/1 -> Add_a5e84/1
  Constant_x_ddd_24bf1/1 -> Divide_23144/2
  Add_c0b37/1 -> Subtract_ceb76/1
  Divide_4a71c/1 -> Subtract_ceb76/2
  State_psi_1d_SG_D_3_a323d/1 -> Product_75d1c/2
  Constant_x_l_16664/1 -> Subtract_178f7/2
  Constant_x_dd_c59a0/1 -> Subtract_eae77/1
  Subtract_c7762/1 -> Product_76ec5/1
  Add_a5e84/1 -> Subtract_06353/1
  Subtract_ceb76/1 -> Product_76ec5/2
  Subtract_eae77/1 -> Product_b3298/2
  Constant_x_dd_60261/1 -> Subtract_49ce1/1
  Constant_x_l_81e97/1 -> Subtract_49ce1/2
  Subtract_45bc0/1 -> Product_1c2f3/2
  Constant_x_dd_f6e51/1 -> Subtract_0d45b/1
  Constant_x_ddd_deeeb/1 -> Subtract_0d45b/2
  Product_eaf90/1 -> Product_7164e/1
  State_psi_1d_SG_D_3_83346/1 -> Subtract_aa4e5/1
  Subtract_49ce1/1 -> Divide_19a64/2
  State_psi_fd_SG_D_3_748b1/1 -> Subtract_aa4e5/2
  Constant_-1_27e1c/1 -> Product_eaf90/1
  Subtract_aa4e5/1 -> Subtract_89049/1
  Divide_23144/1 -> Subtract_89049/2
  Constant_x_dd_2166e/1 -> Subtract_d5f20/1
  Divide_ce65d/1 -> Subtract_06353/2
  State_psi_d_SG_D_3_2010b/1 -> Add_a5e84/2
  Subtract_178f7/1 -> Divide_ce65d/2
  Subtract_89049/1 -> Product_7164e/2
  Subtract_d5f20/1 -> Power_622e4/1
  Constant_2.0_c8f6e/1 -> Power_622e4/2
  Product_7164e/1 -> Divide_d1f36/1
  Subtract_c63d1/1 -> Product_30c76/2
  Power_622e4/1 -> Divide_d1f36/2
  Subtract_06353/1 -> Divide_18b4f/1
  Constant_x_ddd_debb3/1 -> Divide_18b4f/2
  Constant_x_d_61565/1 -> Subtract_48db2/1
  Constant_x_dd_e6636/1 -> Subtract_48db2/2
  Divide_d1f36/1 -> Subtract_c63d1/1
  Divide_18b4f/1 -> Subtract_c63d1/2
  State_E_fd_SG_D_3_c4807/1 -> Subtract_9ff2b/1
  State_psi_fd_SG_D_3_a0d97/1 -> Subtract_9ff2b/2
  Subtract_48db2/1 -> Product_30c76/1
  Subtract_9ff2b/1 -> Subtract_ec1ee/1
  Product_30c76/1 -> Subtract_ec1ee/2
  Subtract_ec1ee/1 -> Divide_55e59/1
  Constant_T_dd_bc5d2/1 -> Divide_55e59/2
  Divide_55e59/1 -> Blockout_d_psi_fd_SG_D_3_350b8/1
